simulink model "byciclemodelsimu"  (R2020a)
settings: Solver=VariableStepAuto  StartTime=0.0  StopTime=15  RelTol=1e-3
undefined symbols (not defined in the file or in its folder): DiscIntNeverNeededParam
libraries: simulink x1
settings Model: Creator=chech  LastModifiedBy=chech

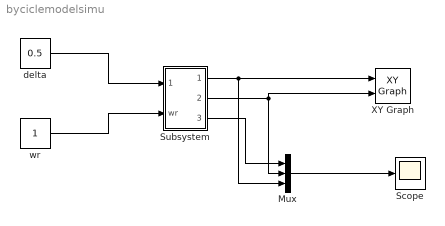
== system byciclemodelsimu ==
  Mux : Mux  Inputs=3
  Scope : Scope
  Subsystem : Subsystem
  XY Graph : simulink/Sinks/XY Graph  xmin=-5  xmax=5  ymin=-5  ymax=5  st=-1
  delta : Constant  Value=0.5
  wr : Constant
  wires:
  Subsystem/1(Out1) -> Mux/3, XY Graph/1
  Subsystem/2(Out2) -> Mux/2, XY Graph/2
  Subsystem/3(Out3) -> Mux/1
  Mux/1 -> Scope/1
  wr/1 -> Subsystem/2(wr)
  delta/1 -> Subsystem/1(delta)

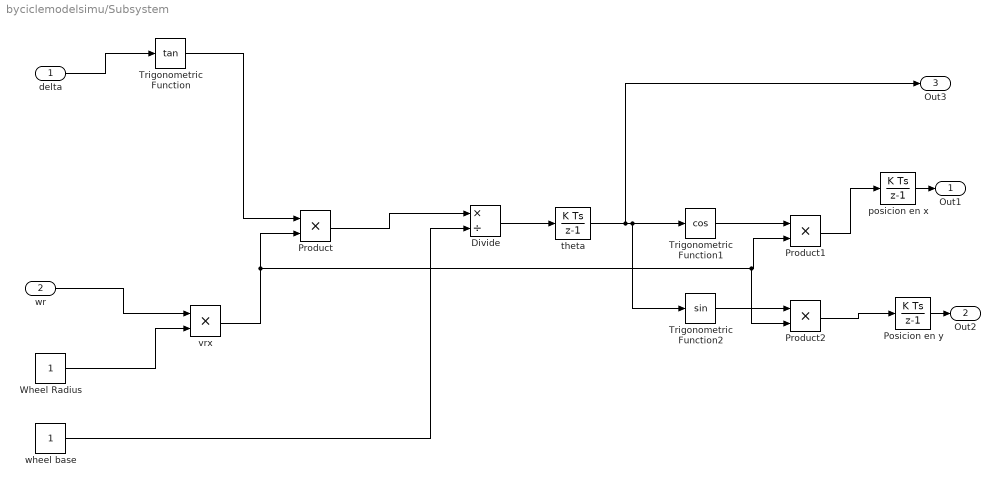
== system byciclemodelsimu/Subsystem ==
  delta : Inport
  wr : Inport  Port=2
  Divide : Product  Inputs=*/
  Posicion en y : DiscreteIntegrator  SampleTime=-1  ICPrevOutput=DiscIntNeverNeededParam  ICPrevScaledInput=DiscIntNeverNeededParam
  Product : Product
  Product1 : Product
  Product2 : Product
  Trigonometric Function : Trigonometry  Operator=tan
  Trigonometric Function1 : Trigonometry  Operator=cos
  Trigonometric Function2 : Trigonometry
  Wheel Radius : Constant
  posicion en x : DiscreteIntegrator  SampleTime=-1  ICPrevOutput=DiscIntNeverNeededParam  ICPrevScaledInput=DiscIntNeverNeededParam
  theta : DiscreteIntegrator  InitialCondition=pi  SampleTime=-1  ICPrevOutput=DiscIntNeverNeededParam  ICPrevScaledInput=DiscIntNeverNeededParam
  vrx : Product
  wheel base : Constant
  Out1 : Outport
  Out2 : Outport  Port=2
  Out3 : Outport  Port=3
  wires:
  Product1/1 -> posicion en x/1
  Product2/1 -> Posicion en y/1
  delta/1 -> Trigonometric Function/1
  Trigonometric Function2/1 -> Product2/1
  theta/1 -> Out3/1, Trigonometric Function2/1, Trigonometric Function1/1
  Divide/1 -> theta/1
  posicion en x/1 -> Out1/1
  Wheel Radius/1 -> vrx/2
  Trigonometric Function/1 -> Product/1
  vrx/1 -> Product2/2, Product1/2, Product/2
  Product/1 -> Divide/1
  Posicion en y/1 -> Out2/1
  wheel base/1 -> Divide/2
  Trigonometric Function1/1 -> Product1/1
  wr/1 -> vrx/1
